simulink model "StateSpaceExe"  (Simulink 7.2)
settings: Solver=ode45  SolverMode=SingleTasking  StartTime=0.0  StopTime=50  RelTol=1e-3
values from neighbouring files (symbols this model uses):
  K = [Kx(1) Kx(2)]    [toStateSpace.m]
  Ki = Kx(3)    [toStateSpace.m]
  L = acker(A', C', [polo1, polo2])'    [toStateSpace.m]
undefined symbols (not defined in the file or in its folder): A, B, C, D
settings Model: Creator=lucas  LastModifiedBy=Aluno  CovMetricSettings=dwe  CovHtmlReporting=off  covSaveCumulativeToWorkspaceVar=off  CovSaveSingleToWorkspaceVar=off
settings DataIOCC: LimitDataPoints=off  SaveFormat=StructureWithTime
settings OptimizationCC: ExpressionDepthLimit=128
settings DebuggingCC: UnderspecifiedInitializationDetection=Simplified  MergeDetectMultiDrivingBlocksExec=error  SolverPrmCheckMsg=none  FcnCallInpInsideContextMsg=Enable All  StateNameClashWarn=none  StrictBusMsg=ErrorLevel1
settings HardwareCC: ProdIntDivRoundTo=Zero  ProdEndianess=LittleEndian  ProdHWDeviceType=Specified
settings SFSimCC: SimUseLocalCustomCode=on
settings RTWCC: RTWUseLocalCustomCode=on
settings CodeAppCC: CustomSymbolStrType=$N$R$M_T
settings GRTTargetCC: TargetFunctionLibrary=C99 (ISO)

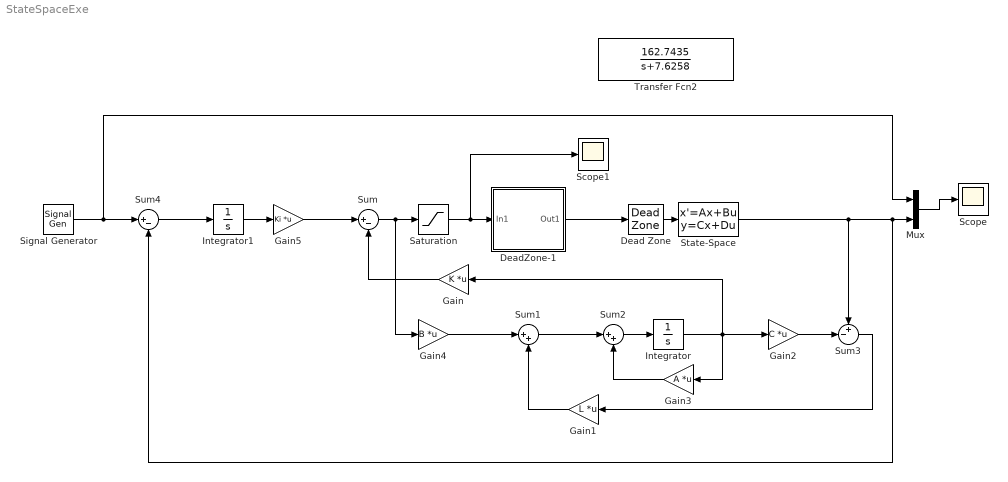
== system StateSpaceExe ==
  Dead Zone : DeadZone  LowerValue=-0.02695  UpperValue=0.5449  ZeroCross=off  SaturateOnIntegerOverflow=on
  DeadZone-1 : Subsystem
  Gain : Gain  Orientation=left  Gain=K  Multiplication=Matrix(K*u)
  Gain1 : Gain  Orientation=left  Gain=L  Multiplication=Matrix(K*u)
  Gain2 : Gain  Gain=C  Multiplication=Matrix(K*u)
  Gain3 : Gain  Orientation=left  Gain=A  Multiplication=Matrix(K*u)
  Gain4 : Gain  Gain=B  Multiplication=Matrix(K*u)
  Gain5 : Gain  Gain=Ki  Multiplication=Matrix(K*u)
  Integrator : Integrator
  Integrator1 : Integrator
  Mux : Mux  Inputs=2
  Saturation : Saturate  UpperLimit=6  LowerLimit=-6
  Scope : Scope
      settings: YMin=150.00389  YMax=243.58992
  Scope1 : Scope
      settings: YMin=-28.32671  YMax=32.53698
  Signal Generator : SignalGenerator  WaveForm=square  Amplitude=200  Frequency=0.1  Units=rad/sec
  State-Space : StateSpace  A=A  B=B  C=C  D=D
  Sum : Sum  Inputs=|+-
  Sum1 : Sum  Inputs=|++
  Sum2 : Sum  Inputs=|++
  Sum3 : Sum  Inputs=+-|
  Sum4 : Sum  Inputs=|+-
  Transfer Fcn2 : TransferFcn  Numerator=[162.7435]  Denominator="[1  7.6258]"
  wires:
  Mux/1 -> Scope/1
  Sum4/1 -> Integrator1/1
  Sum/1 -> Saturation/1, Gain4/1
  Gain2/1 -> Sum3/2
  Gain3/1 -> Sum2/2
  Sum2/1 -> Integrator/1
  Sum3/1 -> Gain1/1
  Gain1/1 -> Sum1/2
  Sum1/1 -> Sum2/1
  Gain4/1 -> Sum1/1
  Integrator/1 -> Gain/1, Gain3/1, Gain2/1
  Gain/1 -> Sum/2
  Signal Generator/1 -> Mux/1, Sum4/1
  Integrator1/1 -> Gain5/1
  Gain5/1 -> Sum/1
  Saturation/1 -> Scope1/1, DeadZone-1/1(In1)
  State-Space/1 -> Sum3/1, Sum4/2, Mux/2
  DeadZone-1/1(Out1) -> Dead Zone/1
  Dead Zone/1 -> State-Space/1

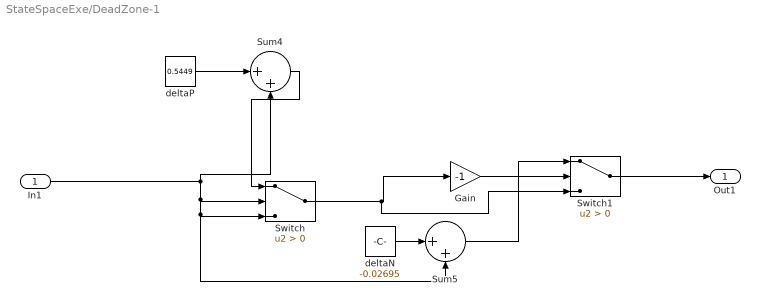
== system StateSpaceExe/DeadZone-1 ==
  In1 : Inport
  Gain : Gain  Gain=-1
  Sum4 : Sum  Inputs=|++
  Sum5 : Sum  Inputs=|++
  Switch : Switch  Criteria=u2 > Threshold
  Switch1 : Switch  Criteria=u2 > Threshold
  deltaN : Constant  Value=-0.02695
  deltaP : Constant  Value=0.5449
  Out1 : Outport
  wires:
  Sum4/1 -> Switch/1
  Switch/1 -> Switch1/3, Gain/1
  Sum5/1 -> Switch1/1
  Gain/1 -> Switch1/2
  deltaN/1 -> Sum5/1
  In1/1 -> Sum4/2, Switch/3, Sum5/2, Switch/2
  Switch1/1 -> Out1/1
  deltaP/1 -> Sum4/1
